simulink model "outerLoop_voltageControl"  (R2024a)
settings: Solver=VariableStepAuto  StartTime=0.0  StopTime=Tsim_outLoop  FixedStep=Tstep  RelTol=1e-3
undefined symbols (not defined in the file): C, den_i, DiscIntNeverNeededParam, ILmax, ILnom, kaw_i, kaw_v, ki_i, ki_v, kp_i, kp_v, kpf_v, num_i, RserC, Tsw, VinNom, VLlim, VoutNom, zden_aaf, zden_pf_v, zden_plant_i, zden_plant_v, znum_aaf, znum_pf_v, znum_plant_i, znum_plant_v
libraries: simulink x3
settings Model: Creator=nicholas  LastModifiedBy=nicholas
settings RTWCC: GPUComputeCapability=3.5

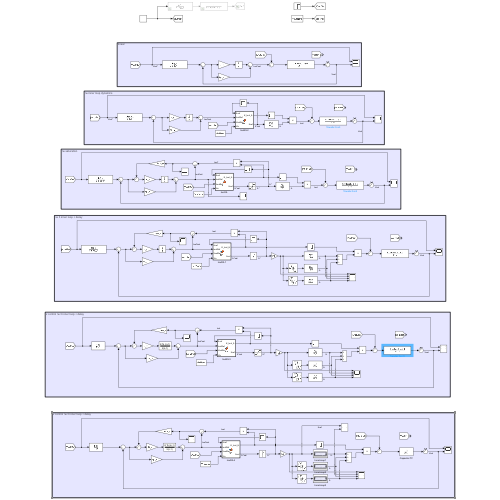
[thumbnail: Simulink's stored preview of the top-level diagram]
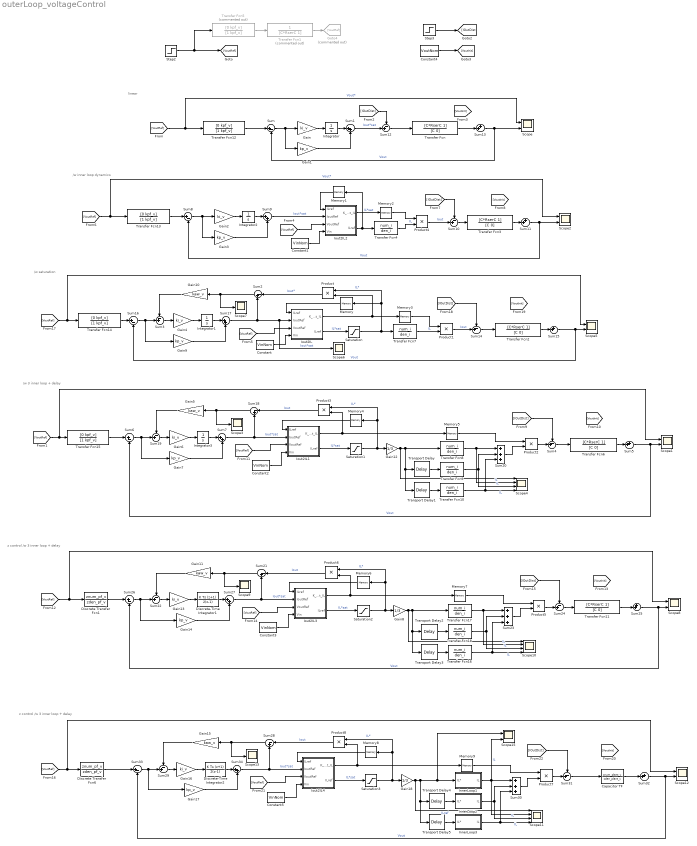
== system outerLoop_voltageControl ==
  note: /w 3 inner loop + delay
  note: /w saturation
  note: /w inner loop dynamics
  note: linear
  note: z control /w 3 inner loop + delay
  note: z control /w 3 inner loop + delay
  Capacitor TF : DiscreteTransferFcn  Numerator=znum_plant_v  Denominator=zden_plant_v
  Constant{,1..3,5} (5 alike) : Constant  Value=VinNom
  Constant4 : Constant  Value=VoutNom
  Discrete Transfer Fcn1 : DiscreteTransferFcn  Numerator=znum_pf_v  Denominator=zden_pf_v
  Discrete Transfer Fcn6 : DiscreteTransferFcn  Numerator=znum_pf_v  Denominator=zden_pf_v
  Discrete-Time Integrator1 : DiscreteIntegrator  IntegratorMethod=Integration: Trapezoidal  SampleTime=Tsw  ICPrevOutput=DiscIntNeverNeededParam  ICPrevScaledInput=DiscIntNeverNeededParam
  Discrete-Time Integrator2 : DiscreteIntegrator  IntegratorMethod=Integration: Trapezoidal  SampleTime=Tsw  ICPrevOutput=DiscIntNeverNeededParam  ICPrevScaledInput=DiscIntNeverNeededParam
  Gain{,2,4,6,13,16} (6 alike) : Gain  Gain=ki_v
  Gain{1,3,7,9,14,17} (6 alike) : Gain  Gain=kp_v
  Gain{5,10..11,15} (4 alike) : Gain  Gain=kaw_v
  Gain12 : Gain  Gain=1/3
  Gain18 : Gain  Gain=1/3
  Gain8 : Gain  Gain=1/3
  Goto4 : Goto  Commented=on  GotoTag=VoutRef
  InnerLoop1 : Subsystem
  InnerLoop2 : Subsystem
  InnerLoop3 : Subsystem
  Integrator{,1..3} (4 alike) : Integrator
  Iout2IL : MATLAB Function  TreatAsAtomicUnit=on
  Iout2IL1 : MATLAB Function  TreatAsAtomicUnit=on
  Iout2IL2 : MATLAB Function  TreatAsAtomicUnit=on
  Iout2IL3 : MATLAB Function  TreatAsAtomicUnit=on
  Iout2IL4 : MATLAB Function  TreatAsAtomicUnit=on
  Memory{,1,4,6,8} (5 alike) : Memory
  Memory{2..3,5,7,9} (5 alike) : Memory  InitialCondition=1
  Product{,1..8} (9 alike) : Product
  Saturation{,1..3} (4 alike) : Saturate  UpperLimit=ILmax  LowerLimit=-ILmax
  Scope{,1..2,5,8,12,15} (7 alike) : Scope  NumInputPorts=2
  Scope10 : Scope  NumInputPorts=4
  Scope11 : Scope  NumInputPorts=4
  Scope{3,6..7,9,13} (5 alike) : Scope
  Scope4 : Scope  NumInputPorts=4
  Step2 : Step  Time=0.1  Before=VinNom  After=VoutNom  SampleTime=0
  Step3 : Step  Time=0.3  After=ILnom/3  SampleTime=0
  Sum{,6,8,16,26,33} (6 alike) : Sum  Inputs=|+-
  Sum{1,7,9,17,27,34} (6 alike) : Sum  Inputs=|++
  Sum{3..4,10,12,14,19,22,24,29,31} (10 alike) : Sum  Inputs=-+|
  Sum{5,11,13,15,25,32} (6 alike) : Sum  Inputs=++|
  Sum{2,18,21,28} (4 alike) : Sum  Inputs=|-+
  Sum20 : Sum  Inputs=+++
  Sum23 : Sum  Inputs=+++
  Sum30 : Sum  Inputs=+++
  Transfer Fcn{,2..3,6,11} (5 alike) : TransferFcn  Numerator=[C*RserC 1]  Denominator=[C 0]
  Transfer Fcn1 : TransferFcn  Commented=on  Denominator=[C*RserC 1]
  Transfer Fcn{4,7..10,16..18} (8 alike) : TransferFcn  Numerator=num_i  Denominator=den_i
  Transfer Fcn{12..15} (4 alike) : TransferFcn  Numerator=[0 kpf_v]  Denominator=[1 kpf_v]
  Transfer Fcn5 : TransferFcn  Commented=on  Numerator=[0 kpf_v]  Denominator=[1 kpf_v]
  Transport Delay : TransportDelay  DelayTime=Tsw/3
  Transport Delay1 : TransportDelay  DelayTime=2*Tsw/3
  Transport Delay2 : TransportDelay  DelayTime=Tsw/3
  Transport Delay3 : TransportDelay  DelayTime=2*Tsw/3
  Transport Delay4 : TransportDelay  DelayTime=Tsw/3
  Transport Delay5 : TransportDelay  DelayTime=2*Tsw/3
  wires:
  [VoutRef] -> Transfer Fcn12/1, Scope/1  "Vout*"
  Gain1/1 -> Sum1/2
  Sum/1 -> Gain/1, Gain1/1
  Gain/1 -> Integrator/1
  Integrator/1 -> Sum1/1
  Sum12/1 -> Transfer Fcn/1
  Step3/1 -> [IOutDist]
  Constant4/1 -> [VoutInit]
  Sum1/1 -> Sum12/2  "Iout*sat"
  Transfer Fcn/1 -> Sum13/2
  Sum13/1 -> Sum/2, Scope/2  "Vout"
  [IOutDist] -> Sum12/1
  Transfer Fcn1/1 -> Goto4/1
  Sum11/1 -> Sum8/2, Scope2/2  "Vout"
  Gain3/1 -> Sum9/2
  Transfer Fcn3/1 -> Sum11/2
  Sum8/1 -> Gain2/1, Gain3/1
  Sum10/1 -> Transfer Fcn3/1
  [VoutRef] -> Transfer Fcn13/1, Scope2/1  "Vout*"
  Integrator2/1 -> Sum9/1
  [IOutDist] -> Sum10/1
  Gain2/1 -> Integrator2/1
  Product1/1 -> Sum14/2  "Iout"
  Gain9/1 -> Sum17/2
  Sum16/1 -> Sum3/2, Gain9/1
  Sum14/1 -> Transfer Fcn2/1
  Transfer Fcn2/1 -> Sum15/2
  Sum15/1 -> Sum16/2, Scope5/2  "Vout"
  [VoutRef] -> Transfer Fcn14/1, Scope5/1
  Sum17/1 -> Sum2/2, Scope6/1, Iout2IL/2(IoutRef)  "Iout*sat"
  Integrator1/1 -> Sum17/1
  Sum3/1 -> Gain4/1
  Iout2IL/1(K_Iout_IL) -> Product/2, Memory3/1
  Memory/1 -> Iout2IL/1("ILref ")
  Constant/1 -> Iout2IL/4(Vin)
  Saturation/1 -> Transfer Fcn7/1, Product/1, Memory/1  "IL*"
  Sum9/1 -> Iout2IL2/2(IoutRef)  "Iout*sat"
  Iout2IL2/2(ILref) -> Memory1/1, Transfer Fcn4/1  "IL*sat"
  Memory1/1 -> Iout2IL2/1("ILref ")
  Constant1/1 -> Iout2IL2/4(Vin)
  [VoutRef] -> Iout2IL2/3(VoutRef)
  Product/1 -> Sum2/1  "Iout*"
  Sum2/1 -> Scope7/1, Gain10/1
  Transfer Fcn4/1 -> Product4/2  "IL"
  Product4/1 -> Sum10/2  "Iout"
  Iout2IL2/1(K_Iout_IL) -> Memory2/1
  Memory2/1 -> Product4/1
  Transfer Fcn7/1 -> Product1/2  "IL"
  Memory3/1 -> Product1/1
  Step2/1 -> [VoutRef], Transfer Fcn5/1
  Gain4/1 -> Integrator1/1
  Gain10/1 -> Sum3/1
  [VoutRef] -> Iout2IL/3(VoutRef)
  Iout2IL/2(ILref) -> Saturation/1  "IL*sat"
  Integrator3/1 -> Sum7/1
  [VoutRef] -> Iout2IL1/3(VoutRef)
  Saturation1/1 -> Product3/1, Memory4/1, Gain12/1  "IL*"
  Gain6/1 -> Integrator3/1
  Sum7/1 -> Iout2IL1/2(IoutRef), Sum18/2  "Iout*sat"
  [IOutDist] -> Sum4/1
  Gain7/1 -> Sum7/2
  Sum4/1 -> Transfer Fcn6/1
  Iout2IL1/2(ILref) -> Saturation1/1  "IL*sat"
  Product2/1 -> Sum4/2
  Memory5/1 -> Product2/1
  Constant2/1 -> Iout2IL1/4(Vin)
  Sum6/1 -> Sum19/2, Gain7/1
  Iout2IL1/1(K_Iout_IL) -> Product3/2, Memory5/1
  Gain5/1 -> Sum19/1
  Sum5/1 -> Sum6/2, Scope1/2  "Vout"
  Sum19/1 -> Gain6/1
  Sum18/1 -> Scope3/1, Gain5/1
  Memory4/1 -> Iout2IL1/1("ILref ")
  [VoutRef] -> Transfer Fcn15/1, Scope1/1
  Transfer Fcn6/1 -> Sum5/2
  Product3/1 -> Sum18/1  "Iout"
  Transport Delay/1 -> Transfer Fcn9/1
  Transport Delay1/1 -> Transfer Fcn10/1
  Gain12/1 -> Scope4/1, Transfer Fcn8/1, Transport Delay/1, Transport Delay1/1
  Transfer Fcn9/1 -> Scope4/3, Sum20/2  "IL"
  Transfer Fcn8/1 -> Scope4/2, Sum20/1  "IL"
  Transfer Fcn10/1 -> Scope4/4, Sum20/3  "IL"
  Sum20/1 -> Product2/2
  [IOutDist] -> Sum14/1
  Gain14/1 -> Sum27/2
  Sum21/1 -> Scope9/1, Gain11/1
  Transport Delay2/1 -> Transfer Fcn18/1
  Sum25/1 -> Sum26/2, Scope8/2  "Vout"
  [VoutRef] -> Discrete Transfer Fcn1/1, Scope8/1
  Transfer Fcn18/1 -> Scope10/3, Sum23/2  "IL"
  Memory6/1 -> Iout2IL3/1("ILref ")
  Sum27/1 -> Iout2IL3/2(IoutRef), Sum21/2  "Iout*sat"
  [VoutRef] -> Iout2IL3/3(VoutRef)
  Gain13/1 -> Discrete-Time Integrator1/1
  Transfer Fcn11/1 -> Sum25/2
  Discrete-Time Integrator1/1 -> Sum27/1
  Gain11/1 -> Sum22/1
  Sum23/1 -> Product5/2
  Sum26/1 -> Sum22/2, Gain14/1
  Constant3/1 -> Iout2IL3/4(Vin)
  Iout2IL3/1(K_Iout_IL) -> Product6/2, Memory7/1
  Sum22/1 -> Gain13/1
  Iout2IL3/2(ILref) -> Saturation2/1  "IL*sat"
  Product5/1 -> Sum24/2
  Memory7/1 -> Product5/1
  [IOutDist] -> Sum24/1
  Product6/1 -> Sum21/1  "Iout"
  Sum24/1 -> Transfer Fcn11/1
  Saturation2/1 -> Product6/1, Memory6/1, Gain8/1  "IL*"
  Transfer Fcn17/1 -> Scope10/2, Sum23/1  "IL"
  Gain8/1 -> Scope10/1, Transfer Fcn17/1, Transport Delay2/1, Transport Delay3/1
  Transport Delay3/1 -> Transfer Fcn16/1
  Transfer Fcn16/1 -> Scope10/4, Sum23/3  "IL"
  InnerLoop1/1(IL) -> Scope15/2, Scope11/2, Sum30/1  "IL"
  Gain16/1 -> Discrete-Time Integrator2/1
  Gain18/1 -> Scope11/1, InnerLoop1/1(IL*), Scope15/1, Transport Delay4/1, Transport Delay5/1  "ILref"
  Discrete-Time Integrator2/1 -> Sum34/1
  Sum31/1 -> Capacitor TF/1
  Iout2IL4/2(ILref) -> Saturation3/1  "IL*sat"
  Constant5/1 -> Iout2IL4/4(Vin)
  [IOutDist] -> Sum31/1
  Sum29/1 -> Gain16/1
  Product7/1 -> Sum31/2
  Transport Delay5/1 -> InnerLoop3/1(IL*)
  Product8/1 -> Sum28/1  "Iout"
  Iout2IL4/1(K_Iout_IL) -> Product8/2, Memory9/1
  Memory9/1 -> Product7/1
  [VoutRef] -> Iout2IL4/3(VoutRef)
  Sum34/1 -> Iout2IL4/2(IoutRef), Sum28/2  "Iout*sat"
  Sum30/1 -> Product7/2
  Sum33/1 -> Sum29/2, Gain17/1
  Capacitor TF/1 -> Sum32/2
  Gain15/1 -> Sum29/1
  InnerLoop3/1(IL) -> Scope11/4, Sum30/3  "IL"
  Memory8/1 -> Iout2IL4/1("ILref ")
  InnerLoop2/1(IL) -> Scope11/3, Sum30/2  "IL"
  Sum28/1 -> Scope13/1, Gain15/1
  Transport Delay4/1 -> InnerLoop2/1(IL*)
  Sum32/1 -> Sum33/2, Scope12/2  "Vout"
  Saturation3/1 -> Product8/1, Memory8/1, Gain18/1  "IL*"
  [VoutRef] -> Scope12/1, Discrete Transfer Fcn6/1
  Gain17/1 -> Sum34/2
  Discrete Transfer Fcn6/1 -> Sum33/1
  Transfer Fcn12/1 -> Sum/1
  Transfer Fcn13/1 -> Sum8/1
  Transfer Fcn14/1 -> Sum16/1
  Transfer Fcn15/1 -> Sum6/1
  Transfer Fcn5/1 -> Transfer Fcn1/1
  Discrete Transfer Fcn1/1 -> Sum26/1

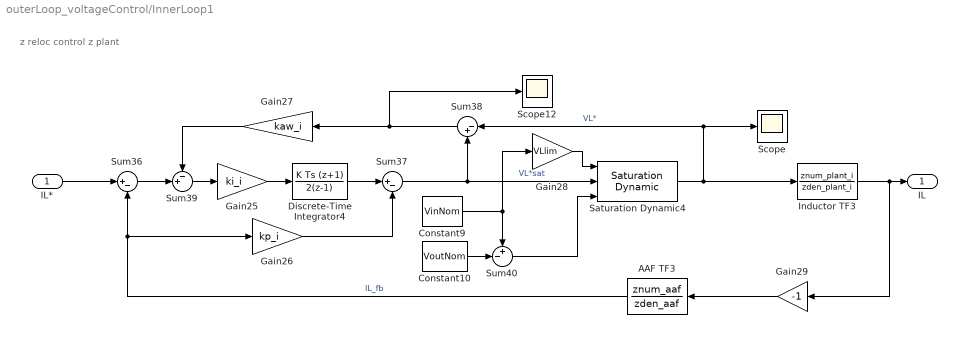
== system outerLoop_voltageControl/InnerLoop1 ==
  note: z reloc control z plant
  IL* : Inport
  AAF TF3 : DiscreteTransferFcn  Numerator=znum_aaf  Denominator=zden_aaf
  Constant10 : Constant  Value=VoutNom
  Constant9 : Constant  Value=VinNom
  Discrete-Time Integrator4 : DiscreteIntegrator  IntegratorMethod=Integration: Trapezoidal  SampleTime=Tsw  ICPrevOutput=DiscIntNeverNeededParam  ICPrevScaledInput=DiscIntNeverNeededParam
  Gain25 : Gain  Gain=ki_i
  Gain26 : Gain  Gain=kp_i
  Gain27 : Gain  Gain=kaw_i
  Gain28 : Gain  Gain=VLlim
  Gain29 : Gain  Gain=-1
  Inductor TF3 : DiscreteTransferFcn  Numerator=znum_plant_i  Denominator=zden_plant_i
  Saturation Dynamic4 : simulink/Discontinuities/Saturation Dynamic  OutMin=[]  OutMax=[]  OutDataTypeStr=Inherit: Same as second input  OutDataType=fixdt(1, 16)  OutScaling=2^-10  DoSatur=off
  Scope : Scope
  Scope12 : Scope
  Sum36 : Sum  Inputs=|+-
  Sum37 : Sum  Inputs=|+-
  Sum38 : Sum  Inputs=|-+
  Sum39 : Sum  Inputs=-+|
  Sum40 : Sum  Inputs=+-|
  IL : Outport
  wires:
  Sum40/1 -> Saturation Dynamic4/3
  Sum37/1 -> Saturation Dynamic4/2, Sum38/2  "VL*sat"
  Saturation Dynamic4/1 -> Inductor TF3/1, Scope/1, Sum38/1  "VL*"
  Sum38/1 -> Gain27/1, Scope12/1
  Sum39/1 -> Gain25/1
  Gain26/1 -> Sum37/2
  Constant10/1 -> Sum40/2
  Discrete-Time Integrator4/1 -> Sum37/1
  Inductor TF3/1 -> Gain29/1, IL/1
  Gain25/1 -> Discrete-Time Integrator4/1
  AAF TF3/1 -> Gain26/1, Sum36/2  "IL_fb"
  Gain29/1 -> AAF TF3/1
  Gain27/1 -> Sum39/1
  Constant9/1 -> Gain28/1, Sum40/1
  Sum36/1 -> Sum39/2
  Gain28/1 -> Saturation Dynamic4/1
  IL*/1 -> Sum36/1

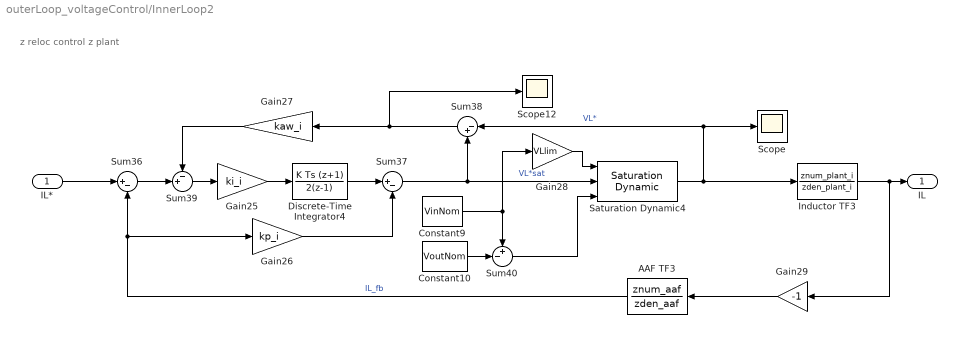
== system outerLoop_voltageControl/InnerLoop2 ==
  note: z reloc control z plant
  IL* : Inport
  AAF TF3 : DiscreteTransferFcn  Numerator=znum_aaf  Denominator=zden_aaf
  Constant10 : Constant  Value=VoutNom
  Constant9 : Constant  Value=VinNom
  Discrete-Time Integrator4 : DiscreteIntegrator  IntegratorMethod=Integration: Trapezoidal  SampleTime=Tsw  ICPrevOutput=DiscIntNeverNeededParam  ICPrevScaledInput=DiscIntNeverNeededParam
  Gain25 : Gain  Gain=ki_i
  Gain26 : Gain  Gain=kp_i
  Gain27 : Gain  Gain=kaw_i
  Gain28 : Gain  Gain=VLlim
  Gain29 : Gain  Gain=-1
  Inductor TF3 : DiscreteTransferFcn  Numerator=znum_plant_i  Denominator=zden_plant_i
  Saturation Dynamic4 : simulink/Discontinuities/Saturation Dynamic  OutMin=[]  OutMax=[]  OutDataTypeStr=Inherit: Same as second input  OutDataType=fixdt(1, 16)  OutScaling=2^-10  DoSatur=off
  Scope : Scope
  Scope12 : Scope
  Sum36 : Sum  Inputs=|+-
  Sum37 : Sum  Inputs=|+-
  Sum38 : Sum  Inputs=|-+
  Sum39 : Sum  Inputs=-+|
  Sum40 : Sum  Inputs=+-|
  IL : Outport
  wires:
  Sum40/1 -> Saturation Dynamic4/3
  Sum37/1 -> Saturation Dynamic4/2, Sum38/2  "VL*sat"
  Saturation Dynamic4/1 -> Inductor TF3/1, Scope/1, Sum38/1  "VL*"
  Sum38/1 -> Gain27/1, Scope12/1
  Sum39/1 -> Gain25/1
  Gain26/1 -> Sum37/2
  Constant10/1 -> Sum40/2
  Discrete-Time Integrator4/1 -> Sum37/1
  Inductor TF3/1 -> Gain29/1, IL/1
  Gain25/1 -> Discrete-Time Integrator4/1
  AAF TF3/1 -> Gain26/1, Sum36/2  "IL_fb"
  Gain29/1 -> AAF TF3/1
  Gain27/1 -> Sum39/1
  Constant9/1 -> Gain28/1, Sum40/1
  Sum36/1 -> Sum39/2
  Gain28/1 -> Saturation Dynamic4/1
  IL*/1 -> Sum36/1

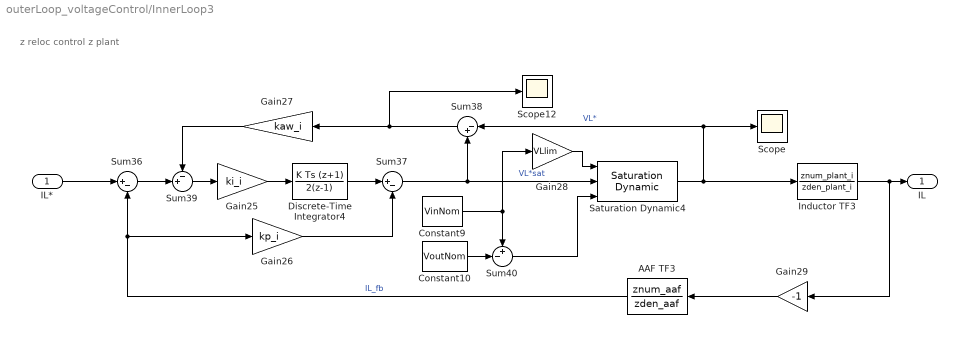
== system outerLoop_voltageControl/InnerLoop3 ==
  note: z reloc control z plant
  IL* : Inport
  AAF TF3 : DiscreteTransferFcn  Numerator=znum_aaf  Denominator=zden_aaf
  Constant10 : Constant  Value=VoutNom
  Constant9 : Constant  Value=VinNom
  Discrete-Time Integrator4 : DiscreteIntegrator  IntegratorMethod=Integration: Trapezoidal  SampleTime=Tsw  ICPrevOutput=DiscIntNeverNeededParam  ICPrevScaledInput=DiscIntNeverNeededParam
  Gain25 : Gain  Gain=ki_i
  Gain26 : Gain  Gain=kp_i
  Gain27 : Gain  Gain=kaw_i
  Gain28 : Gain  Gain=VLlim
  Gain29 : Gain  Gain=-1
  Inductor TF3 : DiscreteTransferFcn  Numerator=znum_plant_i  Denominator=zden_plant_i
  Saturation Dynamic4 : simulink/Discontinuities/Saturation Dynamic  OutMin=[]  OutMax=[]  OutDataTypeStr=Inherit: Same as second input  OutDataType=fixdt(1, 16)  OutScaling=2^-10  DoSatur=off
  Scope : Scope
  Scope12 : Scope
  Sum36 : Sum  Inputs=|+-
  Sum37 : Sum  Inputs=|+-
  Sum38 : Sum  Inputs=|-+
  Sum39 : Sum  Inputs=-+|
  Sum40 : Sum  Inputs=+-|
  IL : Outport
  wires:
  Sum40/1 -> Saturation Dynamic4/3
  Sum37/1 -> Saturation Dynamic4/2, Sum38/2  "VL*sat"
  Saturation Dynamic4/1 -> Inductor TF3/1, Scope/1, Sum38/1  "VL*"
  Sum38/1 -> Gain27/1, Scope12/1
  Sum39/1 -> Gain25/1
  Gain26/1 -> Sum37/2
  Constant10/1 -> Sum40/2
  Discrete-Time Integrator4/1 -> Sum37/1
  Inductor TF3/1 -> Gain29/1, IL/1
  Gain25/1 -> Discrete-Time Integrator4/1
  AAF TF3/1 -> Gain26/1, Sum36/2  "IL_fb"
  Gain29/1 -> AAF TF3/1
  Gain27/1 -> Sum39/1
  Constant9/1 -> Gain28/1, Sum40/1
  Sum36/1 -> Sum39/2
  Gain28/1 -> Saturation Dynamic4/1
  IL*/1 -> Sum36/1

== matlab function outerLoop_voltageControl/Iout2IL1 ==
  data: K_Iout_IL output; ILref input; IoutRef input; VoutRef input; Vin input; ILref output; RserL parameter
function [K_Iout_IL,ILref] = fcn(ILref,IoutRef,VoutRef,Vin,RserL)

if VoutRef < Vin
    VoutRef = Vin;
end
K_Iout_IL = (Vin - RserL*ILref) / VoutRef;
ILref = IoutRef / K_Iout_IL;

== matlab function outerLoop_voltageControl/Iout2IL2 ==
  data: K_Iout_IL output; ILref input; IoutRef input; VoutRef input; Vin input; ILref output; RserL parameter
function [K_Iout_IL,ILref] = fcn(ILref,IoutRef,VoutRef,Vin,RserL)

if VoutRef < Vin
    VoutRef = Vin;
end
K_Iout_IL = (Vin - RserL*ILref) / VoutRef;
ILref = IoutRef / K_Iout_IL;

== matlab function outerLoop_voltageControl/Iout2IL ==
  data: K_Iout_IL output; ILref input; IoutRef input; VoutRef input; Vin input; ILref output; RserL parameter
function [K_Iout_IL,ILref] = fcn(ILref,IoutRef,VoutRef,Vin,RserL)

if VoutRef < Vin
    VoutRef = Vin;
end
K_Iout_IL = (Vin - RserL*ILref) / VoutRef;
ILref = IoutRef / K_Iout_IL;

== matlab function outerLoop_voltageControl/Iout2IL3 ==
  data: K_Iout_IL output; ILref input; IoutRef input; VoutRef input; Vin input; ILref output; RserL parameter
function [K_Iout_IL,ILref] = fcn(ILref,IoutRef,VoutRef,Vin,RserL)

if VoutRef < Vin
    VoutRef = Vin;
end
K_Iout_IL = (Vin - RserL*ILref) / VoutRef;
ILref = IoutRef / K_Iout_IL;

== matlab function outerLoop_voltageControl/Iout2IL4 ==
  data: K_Iout_IL output; ILref input; IoutRef input; VoutRef input; Vin input; ILref output; RserL parameter
function [K_Iout_IL,ILref] = fcn(ILref,IoutRef,VoutRef,Vin,RserL)

if VoutRef < Vin
    VoutRef = Vin;
end
K_Iout_IL = (Vin - RserL*ILref) / VoutRef;
ILref = IoutRef / K_Iout_IL;
